simulink model "simulinkStuff"  (R2023a)
settings: Solver=VariableStepAuto  StartTime=0.0  StopTime=10  RelTol=1e-9
settings Model: Creator=mcconncm  LastModifiedBy=mcconncm

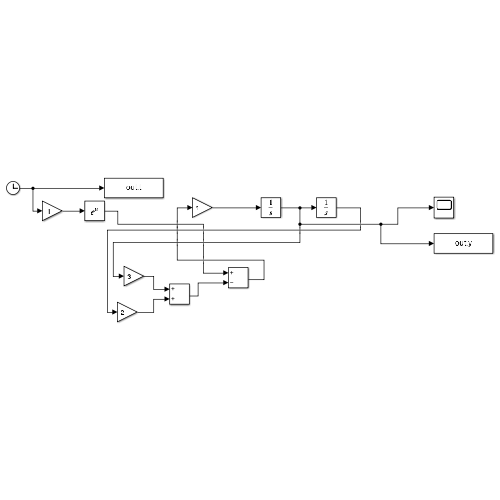
[thumbnail: Simulink's stored preview of the top-level diagram]
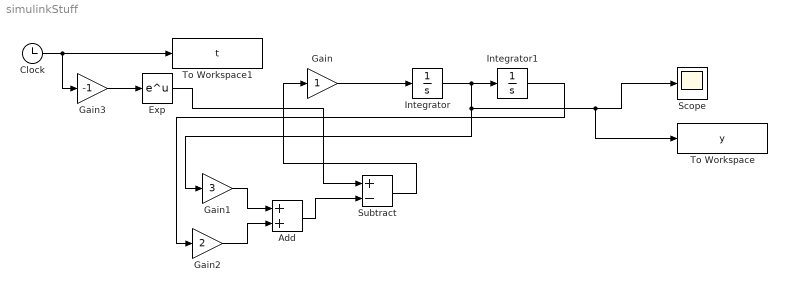
== system simulinkStuff ==
  Add : Sum
  Clock : Clock
  Exp : Math
  Gain : Gain
  Gain1 : Gain  Gain=3
  Gain2 : Gain  Gain=2
  Gain3 : Gain  Gain=-1
  Integrator : Integrator  InitialCondition=.1
  Integrator1 : Integrator  InitialCondition=-.25
  Scope : Scope
  Subtract : Sum  Inputs=+-
  To Workspace : ToWorkspace  VariableName=y  SampleTime=-1
  To Workspace1 : ToWorkspace  VariableName=t  SampleTime=-1
  wires:
  Clock/1 -> Gain3/1, To Workspace1/1
  Gain1/1 -> Add/1
  Add/1 -> Subtract/2
  Gain/1 -> Integrator/1
  Subtract/1 -> Gain/1
  Integrator/1 -> To Workspace/1, Scope/1, Gain1/1, Integrator1/1
  Integrator1/1 -> Gain2/1
  Gain2/1 -> Add/2
  Exp/1 -> Subtract/1
  Gain3/1 -> Exp/1
